simulink model "Optical_Movement_Detection_PAR"  (Simulink 7.5)
settings: Solver=ode45  StartTime=0.0  StopTime=inf  RelTol=1e-3
values from neighbouring files (symbols this model uses):
  D = 1    [Copter_Animation.m]
  HSE_Bottom_1 = imresize(imread('D:\GoogleMapsBilder\PAR\HSE_Bottom_1.jpg'), 1)    [TESTS_Optical_Flow_Scenarios.m]
undefined symbols (not defined in the file or in its folder): fspecial, Kanade, Low, Lucas, Rec, SDTV
libraries: simulink x13, dspobslib x10, vipgeotforms x3, vipanalysis x3, dspstat3 x3, dspmtrx3 x2, dspsigops x2, vipconversions x1, dspswit3 x1, vipsrcs x1, viptextngfix x1, vipsnks x1
(part 2 of 2)

== system Optical_Movement_Detection_PAR/Image Processing/Optical Flow/Corner Matching/Calculate Distances/For Iterator Subsystem/For Iterator Subsystem ==
  F1 : Inport  OutDataType=sfix(16)  OutScaling=2^0
  N1 : Inport  Port=2  OutDataType=sfix(16)  OutScaling=2^0
  f2 : Inport  Port=3  OutDataType=sfix(16)  OutScaling=2^0
  Distance between two feature vectors : Subsystem
  For Iterator : ForIterator  IterationSource=external  IndexMode=Zero-based
  Select feature  for 1 corner : Selector  NumberOfDimensions=2  IndexMode=Zero-based  InputPortWidth=2  IndexOptions=Select all,Index vector (port)  Indices=0,1  OutputSizes=1,1
  Update feature  for a corner : Assignment  NumberOfDimensions=2  IndexMode=Zero-based  OutputInitialize=Specify size for each dimension in table  IndexOptions=Index vector (port),Assign all  Indices=1,1  OutputSizes=maxNum,1
  Dis : Outport  OutDataType=sfix(16)  OutScaling=2^0
  wires:
  Select feature  for 1 corner/1 -> Distance between two feature vectors/1(f1)
  f2/1 -> Distance between two feature vectors/2(f2)
  Update feature  for a corner/1 -> Dis/1
  F1/1 -> Select feature  for 1 corner/1
  For Iterator/1 -> Select feature  for 1 corner/2, Update feature  for a corner/2
  N1/1 -> For Iterator/1
  Distance between two feature vectors/1(dis) -> Update feature  for a corner/1

== system Optical_Movement_Detection_PAR/Image Processing/Optical Flow/Corner Matching/Calculate Features/Clip Point Coordinates/Clip row/col coordinates ==
  Low : Inport  OutDataType=sfix(16)  OutScaling=2^0
  High : Inport  Port=2  OutDataType=sfix(16)  OutScaling=2^0
  Coordinates : Inport  Port=3
  Num : Inport  Port=4  OutDataType=sfix(16)  OutScaling=2^0
  Clip a Coordinate : Subsystem
  For Iterator : ForIterator  IterationSource=external  IterationLimit=2  IndexMode=Zero-based
  Select Coordinate of a Point : Selector  NumberOfDimensions=2  IndexMode=Zero-based  InputPortWidth=3  IndexOptions=Select all,Index vector (port)  Indices=[1 3],1  OutputSizes=9,1
  Update Feature  for a Corner : Assignment  NumberOfDimensions=2  IndexMode=Zero-based  IndexOptions=Assign all,Index vector (port)  Indices=1,1  OutputSizes=81,50
  Coordinates_clip : Outport  OutDataType=sfix(16)  OutScaling=2^0
  wires:
  Clip a Coordinate/1(Coordinate_clip) -> Update Feature  for a Corner/2
  Update Feature  for a Corner/1 -> Coordinates_clip/1
  High/1 -> Clip a Coordinate/2(High)
  Low/1 -> Clip a Coordinate/1(Low)
  Select Coordinate of a Point/1 -> Clip a Coordinate/3(Coordinate)
  Num/1 -> For Iterator/1
  Coordinates/1 -> Update Feature  for a Corner/1, Select Coordinate of a Point/1
  For Iterator/1 -> Select Coordinate of a Point/2, Update Feature  for a Corner/3

== system Optical_Movement_Detection_PAR/Image Processing/Optical Flow/Corner Matching/Calculate Distances/For Iterator Subsystem/For Iterator Subsystem/Distance between two feature vectors ==
  f1 : Inport  OutDataType=sfix(16)  OutScaling=2^0
  f2 : Inport  Port=2  OutDataType=sfix(16)  OutScaling=2^0
  Abs : Abs  OutDataType=sfix(16)  OutScaling=2^0
  Add : Sum  Inputs=+-  OutDataType=sfix(16)  OutScaling=2^-10
  Sum of Elements : Sum  Inputs=+  OutDataType=sfix(16)  OutScaling=2^-10
  dis : Outport  OutDataType=sfix(16)  OutScaling=2^0
  wires:
  Sum of Elements/1 -> dis/1
  Abs/1 -> Sum of Elements/1
  Add/1 -> Abs/1
  f2/1 -> Add/2
  f1/1 -> Add/1

== system Optical_Movement_Detection_PAR/Image Processing/Optical Flow/Corner Matching/Calculate Features/Clip Point Coordinates/Clip row/col coordinates/Clip a Coordinate ==
  Low : Inport  OutDataType=sfix(16)  OutScaling=2^0
  High : Inport  Port=2  OutDataType=sfix(16)  OutScaling=2^0
  Coordinate : Inport  Port=3  OutDataType=sfix(16)  OutScaling=2^0
  MinMax1 : MinMax  Function=max  Inputs=2  OutDataType=sfix(16)  OutScaling=2^0
  MinMax2 : MinMax  Inputs=2  OutDataType=sfix(16)  OutScaling=2^0
  Coordinate_clip : Outport  OutDataType=sfix(16)  OutScaling=2^0
  wires:
  MinMax2/1 -> Coordinate_clip/1
  High/1 -> MinMax2/2
  MinMax1/1 -> MinMax2/1
  Low/1 -> MinMax1/2
  Coordinate/1 -> MinMax1/1

== matlab function Image Processing/Optical Flow/Optical Flow Segmentation in Sectors/Optical Flow Lines1 ==
  data: vel_Values input double; Cam_Img_Dim input double; vel_Lines output double; Omega_avg output double; scaleFactor parameter double size=1
function [vel_Lines, Omega_avg]=OpticalFlowLines(vel_Values, Cam_Img_Dim,scaleFactor) 

% Generates the coordinate points of optical flow lines

persistent first_time;
persistent X;
persistent Y;
persistent RV;
persistent CV;

%persistent Max_Vec_Length;

persistent Origin_Re;
persistent Origin_Im;

persistent Sec_1_Cnt;
persistent Sec_2_Cnt;
persistent Sec_3_Cnt;
persistent Sec_4_Cnt;

persistent Sec_1;
persistent Sec_2;
persistent Sec_3;
persistent Sec_4;

persistent R;
persistent C;
persistent Test_mat;
persistent med_vel_val;

%med_vel_val=median(vel_Values);
%[R C] = size(med_vel_val);
if isempty(first_time)
    first_time     = 1;
    Origin_Re = Cam_Img_Dim(1)/2%double(176);
    [R C] = size(vel_Values)
    Origin_Im = Cam_Img_Dim(2)/2%double(144);
end

Sec_1 = double(0);
Sec_2 = double(0);
Sec_3 = double(0);
Sec_4 = double(0);

Sec_1_Cnt = 1;
Sec_2_Cnt = 1;
Sec_3_Cnt = 1;
Sec_4_Cnt = 1;

%sectors
%       ^Im
%       |         
%   4   |  1
%-------------->Re
%   3   |  2
%       |

% for i=1:R
%     for k=1:C
%       j=vel_Values(i,k);
%     if(real(j)>=0) % Sec_1 or Sec_2
%         if(imag(j)>=0) %Sec_1
%             Sec_1_Cnt=Sec_1_Cnt+1;
%             Sec_1=Sec_1+double(abs(j))
%         else           %Sec_2
%             Sec_2_Cnt=Sec_2_Cnt+1;
%             Sec_2=Sec_2+double(abs(j))
%         end
%     else            % Sec_3 or Sec_4
%         if(imag(j)>=0) %Sec_4
%             Sec_4_Cnt=Sec_4_Cnt+1;
%             Sec_4=Sec_4+double(abs(j))
%         else           %Sec_3
%             Sec_3_Cnt=Sec_3_Cnt+1;
%             Sec_3=Sec_3+double(abs(j))
%         end
%     end
%     end
% end

%Other segm
for i=1:R
    for k=1:C
      j=vel_Values(i,k);
    if(real(j)>=0) % Sec_1 or Sec_2
        Sec_1_Cnt=Sec_1_Cnt+1;
        Sec_1=Sec_1+double(abs(real(j)));
        if(imag(j)>=0) %Sec_2
            Sec_2_Cnt=Sec_2_Cnt+1;
            Sec_2=Sec_2+double(imag(j));
        else           %Sec_4
            Sec_4_Cnt=Sec_4_Cnt+1;
            Sec_4=Sec_4+double(imag(j));
        end
    else            % Sec_3 or Sec_4
        Sec_3_Cnt=Sec_3_Cnt+1;
        Sec_3=Sec_3+double(abs(real(j)));
        if(imag(j)>=0) %Sec_2
            Sec_2_Cnt=Sec_2_Cnt+1;
            Sec_2=Sec_2+double(imag(j));
        else           %Sec_4
            Sec_4_Cnt=Sec_4_Cnt+1;
            Sec_4=Sec_4+double(imag(j));
        end
    end
    end
end


% Sec_1_Mat = vel_Values((real(vel_Values) >= 0) & (imag(vel_Values) >= 0));
% Sec_2_Mat = vel_Values((real(vel_Values) >= 0) & (imag(vel_Values) < 0));
% Sec_3_Mat = vel_Values((real(vel_Values) < 0) & (imag(vel_Values) < 0));
% Sec_4_Mat = vel_Values((real(vel_Values) < 0) & (imag(vel_Values) >= 0));


% Sec_1 = sum(abs(Sec_1_Mat)/(size(Sec_1_Mat, 1)*size(Sec_1_Mat, 2)));
% Sec_2 = sum(abs(Sec_1_Mat)/(size(Sec_1_Mat, 1)*size(Sec_1_Mat, 2)));
% Sec_3 = sum(abs(Sec_1_Mat)/(size(Sec_1_Mat, 1)*size(Sec_1_Mat, 2)));
% Sec_4 = sum(abs(Sec_1_Mat)/(size(Sec_1_Mat, 1)*size(Sec_1_Mat, 2)));

Sec_1 = Sec_1/Sec_1_Cnt;
Sec_2 = Sec_2/Sec_2_Cnt;
Sec_3 = Sec_3/Sec_3_Cnt;
Sec_4 = Sec_4/Sec_4_Cnt;

% Omega_Re_Plus = (scaleFactor*(Sec_1+Sec_2))/2
% Omega_Re_Minus = (scaleFactor*(Sec_3+Sec_4))/2
% Omega_Im_Plus = (scaleFactor*(Sec_1+Sec_4))/2
% Omega_Im_Minus = (scaleFactor*(Sec_3+Sec_2))/2

Omega_Re_Plus = scaleFactor*Sec_1; %Sec_2
Omega_Re_Minus = scaleFactor*Sec_3; %Sec_4
Omega_Im_Plus = scaleFactor*Sec_4; %Sec_1
Omega_Im_Minus = scaleFactor*Sec_2; %Sec_3

%Calculation of rotation

rotation_comp=min([abs(Omega_Re_Plus) abs(Omega_Re_Minus) abs(Omega_Im_Plus) abs(Omega_Im_Minus)]);

if(rotation_comp>0)
    Omega_avg = [abs(Omega_Re_Plus)-rotation_comp abs(Omega_Re_Minus)-rotation_comp abs(Omega_Im_Plus)-rotation_comp abs(Omega_Im_Minus)-rotation_comp rotation_comp];
else
    Omega_avg = [abs(Omega_Re_Plus) abs(Omega_Re_Minus) abs(Omega_Im_Plus) abs(Omega_Im_Minus) rotation_comp];
end


vel_Lines = [[Origin_Im Origin_Im Origin_Im Origin_Im];[Origin_Re Origin_Re Origin_Re Origin_Re];...
[Origin_Im Origin_Im+abs(Omega_Im_Minus) Origin_Im Origin_Im-abs(Omega_Im_Plus)];[Origin_Re+abs(Omega_Re_Plus) Origin_Re Origin_Re-abs(Omega_Re_Minus) Origin_Re]];

== matlab function Image Processing/Optical Flow/Cross for callibration/Optical Flow Lines1 ==
  data: vel_Values input double; Cam_Img_Dim input double; vel_Lines output double
function vel_Lines =OpticalFlowLines(vel_Values, Cam_Img_Dim) 

% Generates the coordinate points of optical flow lines

persistent first_time;
persistent X;
persistent Y;
persistent RV;
persistent CV;

%persistent Max_Vec_Length;

persistent Origin_Re;
persistent Origin_Im;

persistent Sec_1_Cnt;
persistent Sec_2_Cnt;
persistent Sec_3_Cnt;
persistent Sec_4_Cnt;

persistent Sec_1;
persistent Sec_2;
persistent Sec_3;
persistent Sec_4;

persistent R;
persistent C;
persistent Test_mat;
persistent med_vel_val;

%med_vel_val=median(vel_Values);
%[R C] = size(med_vel_val);
if isempty(first_time)
    first_time     = 1;
    Origin_Re = Cam_Img_Dim(1)/2%double(176);
    [R C] = size(vel_Values)
    Origin_Im = Cam_Img_Dim(2)/2%double(144);
end


Omega_Re_Plus = 700;
Omega_Re_Minus = 700;
Omega_Im_Plus = 700;
Omega_Im_Minus = 700;


vel_Lines = [[Origin_Im Origin_Im Origin_Im Origin_Im];[Origin_Re Origin_Re Origin_Re Origin_Re];...
[Origin_Im Origin_Im+abs(Omega_Im_Minus) Origin_Im Origin_Im-abs(Omega_Im_Plus)];[Origin_Re+abs(Omega_Re_Plus) Origin_Re Origin_Re-abs(Omega_Re_Minus) Origin_Re]];

== matlab function Image Processing/Optical Flow/Embedded MATLAB Function ==
  data: Pts1 input double; vec output double; Tform input double
function vec = clc(Pts1, Tform)
%#eml

vec=complex(sum(inv(Tform)*Pts1))

== matlab function Image Processing/Optical Flow/Optical Flow Lines1/Optical Flow Lines1 ==
  data: vel_Values input double; vel_Lines output double; dir_Vec output double; scaleFactor parameter double size=1
function [vel_Lines, dir_Vec]=OpticalFlowLines(vel_Values, scaleFactor) 

% Generates the coordinate points of optical flow lines

persistent first_time;
persistent X;
persistent Y;
persistent RV;
persistent CV;
if isempty(first_time)
    first_time     = 1;
    %% user may change the following three parameters
    borderOffset   = 5;
    decimFactorRow = 5;
    decimFactorCol = 5;    
    %%
    [R C] = size(vel_Values);
    RV = borderOffset:decimFactorRow:(R-borderOffset);   
    CV = borderOffset:decimFactorCol:(C-borderOffset);
    [Y X] = meshgrid(CV,RV);
end

tmp = vel_Values(RV,CV);
tmp = tmp.*(-1);
X(:)=180;Y(:)=180;
tmp=sum(tmp(:))/size(tmp(:), 2);
dir_Vec = scaleFactor*[real(tmp), imag(tmp)];
vel_Lines = [X(:)';Y(:)';X(:)'+imag(tmp(:))';Y(:)'+real(tmp(:))'];

== matlab function Image Processing/Optical Flow/Optical Flow Lines2/Optical Flow Lines1 ==
  data: vel_Values input double; vel_Lines output double; dir_Vec output double; scaleFactor parameter double size=1
function [vel_Lines, dir_Vec]=OpticalFlowLines(vel_Values, scaleFactor) 

% Generates the coordinate points of optical flow lines

persistent first_time;
persistent X;
persistent Y;
persistent RV;
persistent CV;
if isempty(first_time)
    first_time     = 1;
    %% user may change the following three parameters
    borderOffset   = 5;
    decimFactorRow = 5;
    decimFactorCol = 5;    
    %%
    [R C] = size(vel_Values);
    RV = borderOffset:decimFactorRow:(R-borderOffset);   
    CV = borderOffset:decimFactorCol:(C-borderOffset);
    [Y X] = meshgrid(CV,RV);
end

tmp = vel_Values(RV,CV);
tmp = tmp.*scaleFactor;
dir_Vec = scaleFactor*[real(tmp), imag(tmp)];
vel_Lines = [X(:)';Y(:)';X(:)'+imag(tmp(:))';Y(:)'+real(tmp(:))'];
